simulink model "Model_sim"  (R2016a)
settings: Solver=VariableStepAuto  StartTime=0.0  StopTime=model.Tsim  MaxStep=1/model.fs  RelTol=1e-3
undefined symbols (not defined in the file or in its folder): DLchar, model, sensor
settings Model: Creator=Marcin  LastModifiedBy=Marcin
settings GRTTargetCC: GeneratePreprocessorConditionals=Use local settings

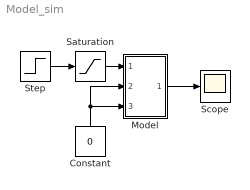
== system Model_sim ==
  Constant : Constant  Value=0
  Model : Subsystem
  Saturation : Saturate  UpperLimit=1  LowerLimit=0
  Scope : Scope
  Step : Step  SampleTime=0
  wires:
  Constant/1 -> Model/3(z2(t)), Model/2(z1(t))
  Model/1(y(t)) -> Scope/1
  Step/1 -> Saturation/1
  Saturation/1 -> Model/1(u(t))

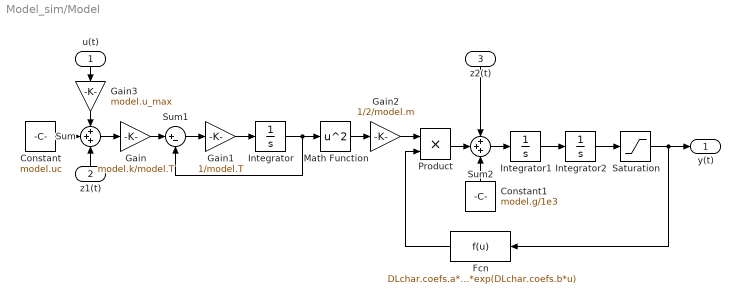
== system Model_sim/Model ==
  u(t) : Inport
  z1(t) : Inport  Port=2
  z2(t) : Inport  Port=3
  Constant : Constant  Value=model.uc
  Constant1 : Constant  Value=model.g/1e3
  Fcn : Fcn  Expr=DLchar.coefs.a*DLchar.coefs.b*exp(DLchar.coefs.b*u)
  Gain : Gain  Gain=model.k/model.T
  Gain1 : Gain  Gain=1/model.T
  Gain2 : Gain  Gain=1/2/model.m
  Gain3 : Gain  Gain=model.u_max
  Integrator : Integrator
  Integrator1 : Integrator
  Integrator2 : Integrator
  Math Function : Math  Operator=square  SaturateOnIntegerOverflow=on
  Product : Product
  Saturation : Saturate  UpperLimit=sensor.d(end)  LowerLimit=sensor.d(1)
  Sum : Sum  Inputs=+++
  Sum1 : Sum  Inputs=|+-
  Sum2 : Sum  Inputs=+++
  y(t) : Outport
  wires:
  Constant/1 -> Sum/2
  Sum/1 -> Gain/1
  z1(t)/1 -> Sum/3
  Gain/1 -> Sum1/1
  Sum1/1 -> Gain1/1
  Gain1/1 -> Integrator/1
  Integrator/1 -> Math Function/1, Sum1/2
  Math Function/1 -> Gain2/1
  Gain2/1 -> Product/1
  Product/1 -> Sum2/2
  z2(t)/1 -> Sum2/1
  Constant1/1 -> Sum2/3
  Sum2/1 -> Integrator1/1
  Integrator1/1 -> Integrator2/1
  Integrator2/1 -> Saturation/1
  Saturation/1 -> y(t)/1, Fcn/1
  Fcn/1 -> Product/2
  u(t)/1 -> Gain3/1
  Gain3/1 -> Sum/1
